simulink model "DSOGI"  (R2018b)
settings: Solver=ode45  StartTime=0.0  StopTime=10.0  MaxStep=0.0001  MinStep=0.00001  RelTol=1e-3
libraries: simulink x1, powerlib_meascontrol x1, powerlib x1
settings Model: Creator=lokes  LastModifiedBy=lokes

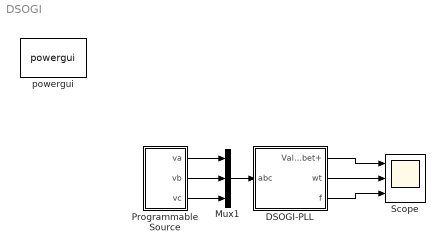
== system DSOGI ==
  DSOGI-PLL : Subsystem
  Mux1 : Mux  Inputs=3
  Programmable Source : Subsystem  mask(DSOGI - PLL){f=50, V=230}
      mask prompts: f "Fundamental grid frequency (f) in Hz"; V "Fundamental grid voltage (V) in RMS volts"
      mask help: Programmable source generates a signal with fundamental and odd harmonic signals upto 13th frequency component.
  Scope : Scope  NumInputPorts=3
  powergui : powerlib/powergui  Priority=1  SimulationMode=Discrete  SampleTime=10e-6  frequency=60  Iterations=50  frequencyindice=60  Pbase=100e6  ErrMax=1e-4  UnitsV=kV  UnitsW=MW  buscounter=0  FunctionMessages=off  echomessages=off  EnableUseOfTLC=off  CurrentSourceSwitches=off  DisableSnubberDevices=off  DisableRonSwitches=off  DisableVfSwitches=off  DisplayEquations=off  SolverType=Tustin/Backward Euler (TBE)  Interpol=off  ExternalGateDelay=off  methode=off  Ts=100  x0status=blocks  SPID=off  SwTol=0  HookPort=off  RestoreLinks=warning  ResistiveCurrentMeasurement=off  Frange=[0:2:500]  Ylog=off  Xlog=on  ShowGrid=off  save=off  variable=ZData  structure=0  ZoomFFT=off  StartTime=0.0  cycles=1  DisplayStyle=1  fundamental=60  FreqAxis=off  MaxFrequency=1000  frequencyindicesteady=1  RmsSteady=1  display=off
  wires:
  Mux1/1 -> DSOGI-PLL/1(abc)
  Programmable Source/1(va) -> Mux1/1
  Programmable Source/2(vb) -> Mux1/2
  Programmable Source/3(vc) -> Mux1/3
  DSOGI-PLL/1(Valp_bet+) -> Scope/1
  DSOGI-PLL/2(wt) -> Scope/2
  DSOGI-PLL/3(f) -> Scope/3

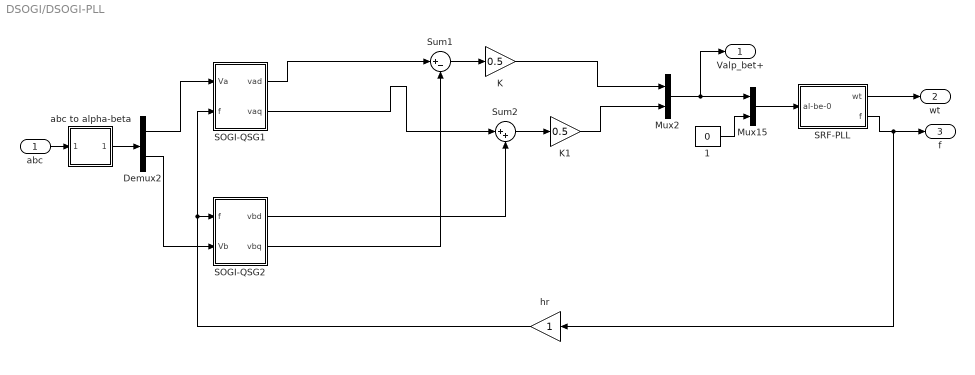
== system DSOGI/DSOGI-PLL ==
  abc : Inport
  1 : Constant  Value=0
  Demux2 : Demux  Outputs=2
  K : Gain  Gain=0.5
  K1 : Gain  Gain=0.5
  Mux15 : Mux  Inputs=2
  Mux2 : Mux  Inputs=2
  SOGI-QSG1 : Subsystem
  SOGI-QSG2 : Subsystem
  SRF-PLL : Subsystem
  Sum1 : Sum  Inputs=|+-
  Sum2 : Sum  Inputs=|++
  abc to alpha-beta : Subsystem
      mask Display:
      | plot([0 1], [0,1])
      | text(0.15,0.7,'abc')
      | text(0.55, 0.3,'\alpha\beta','texmode','on')
  hr : Gain
  Valp_bet+ : Outport
  wt : Outport  Port=2
  f : Outport  Port=3
  wires:
  abc/1 -> abc to alpha-beta/1(abc)
  SOGI-QSG1/1(vad) -> Sum1/1
  Demux2/1 -> SOGI-QSG1/1(Va)
  abc to alpha-beta/1(al_be) -> Demux2/1
  Demux2/2 -> SOGI-QSG2/2(Vb)
  SOGI-QSG2/1(vbd) -> Sum2/2
  SOGI-QSG2/2(vbq) -> Sum1/2
  Sum1/1 -> K/1
  K/1 -> Mux2/1
  SOGI-QSG1/2(vaq) -> Sum2/1
  Sum2/1 -> K1/1
  K1/1 -> Mux2/2
  SRF-PLL/1(wt) -> wt/1
  SRF-PLL/2(f) -> hr/1, f/1
  Mux15/1 -> SRF-PLL/1(al-be-0)
  1/1 -> Mux15/2
  Mux2/1 -> Valp_bet+/1, Mux15/1
  hr/1 -> SOGI-QSG1/2(f), SOGI-QSG2/1(f)

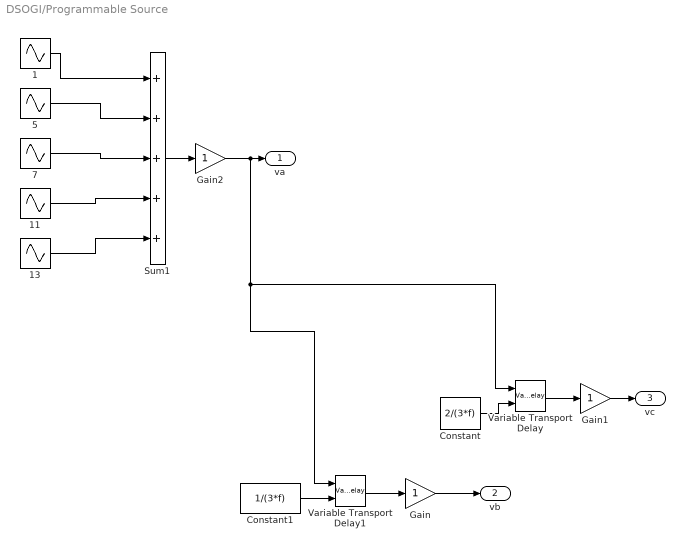
== system DSOGI/Programmable Source ==
  1 : Sin  Amplitude=V*sqrt(2)  Frequency=2*pi*f  Phase=0*pi/2  SampleTime=0
  11 : Sin  Amplitude=V*sqrt(2)/11  Frequency=2*pi*11*f  Phase=0*pi/2  SampleTime=0
  13 : Sin  Amplitude=V*sqrt(2)/13  Frequency=2*pi*13*f  Phase=0*pi/2  SampleTime=0
  5 : Sin  Amplitude=V*sqrt(2)/5  Frequency=2*pi*5*f  Phase=0*pi/2  SampleTime=0
  7 : Sin  Amplitude=V*sqrt(2)/7  Frequency=2*pi*7*f  Phase=0*pi/2  SampleTime=0
  Constant : Constant  Value=2/(3*f)
  Constant1 : Constant  Value=1/(3*f)
  Gain : Gain
  Gain1 : Gain
  Gain2 : Gain
  Sum1 : Sum  Inputs=+++++
  Variable Transport Delay : VariableTransportDelay  VariableDelayType=Variable transport delay  MaximumDelay=10
  Variable Transport Delay1 : VariableTransportDelay  VariableDelayType=Variable transport delay  MaximumDelay=10
  va : Outport
  vb : Outport  Port=2
  vc : Outport  Port=3
  wires:
  Constant1/1 -> Variable Transport Delay1/2
  Constant/1 -> Variable Transport Delay/2
  Variable Transport Delay1/1 -> Gain/1
  Variable Transport Delay/1 -> Gain1/1
  Gain/1 -> vb/1
  Gain1/1 -> vc/1
  Sum1/1 -> Gain2/1
  Gain2/1 -> Variable Transport Delay1/1, Variable Transport Delay/1, va/1
  1/1 -> Sum1/1
  5/1 -> Sum1/2
  7/1 -> Sum1/3
  11/1 -> Sum1/4
  13/1 -> Sum1/5

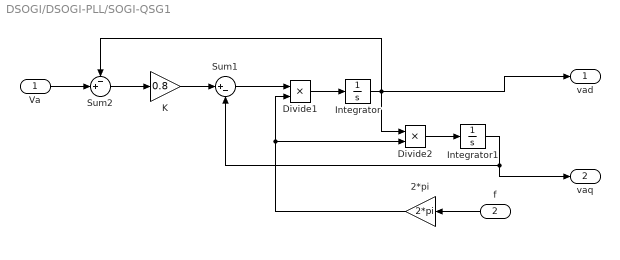
== system DSOGI/DSOGI-PLL/SOGI-QSG1 ==
  Va : Inport
  f : Inport  Port=2
  2*pi : Gain  Gain=2*pi
  Divide1 : Product  Inputs=**
  Divide2 : Product  Inputs=**
  Integrator : Integrator
  Integrator1 : Integrator
  K : Gain  Gain=0.8
  Sum1 : Sum  Inputs=|+-
  Sum2 : Sum  Inputs=-+|
  vad : Outport
  vaq : Outport  Port=2
  wires:
  2*pi/1 -> Divide1/2, Divide2/2
  Va/1 -> Sum2/2
  Integrator1/1 -> vaq/1, Sum1/2
  Divide2/1 -> Integrator1/1
  Integrator/1 -> vad/1, Divide2/1, Sum2/1
  Sum2/1 -> K/1
  K/1 -> Sum1/1
  Sum1/1 -> Divide1/1
  Divide1/1 -> Integrator/1
  f/1 -> 2*pi/1

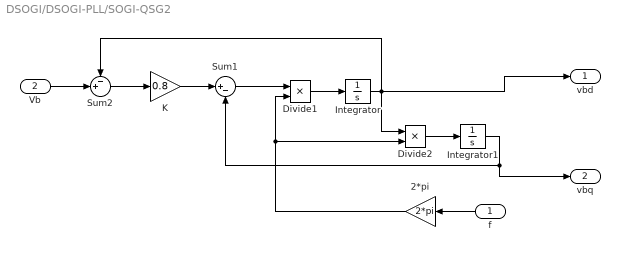
== system DSOGI/DSOGI-PLL/SOGI-QSG2 ==
  f : Inport
  Vb : Inport  Port=2
  2*pi : Gain  Gain=2*pi
  Divide1 : Product  Inputs=**
  Divide2 : Product  Inputs=**
  Integrator : Integrator
  Integrator1 : Integrator
  K : Gain  Gain=0.8
  Sum1 : Sum  Inputs=|+-
  Sum2 : Sum  Inputs=-+|
  vbd : Outport
  vbq : Outport  Port=2
  wires:
  Divide1/1 -> Integrator/1
  Sum1/1 -> Divide1/1
  K/1 -> Sum1/1
  Sum2/1 -> K/1
  Integrator/1 -> Sum2/1, Divide2/1, vbd/1
  Divide2/1 -> Integrator1/1
  Integrator1/1 -> Sum1/2, vbq/1
  Vb/1 -> Sum2/2
  2*pi/1 -> Divide2/2, Divide1/2
  f/1 -> 2*pi/1

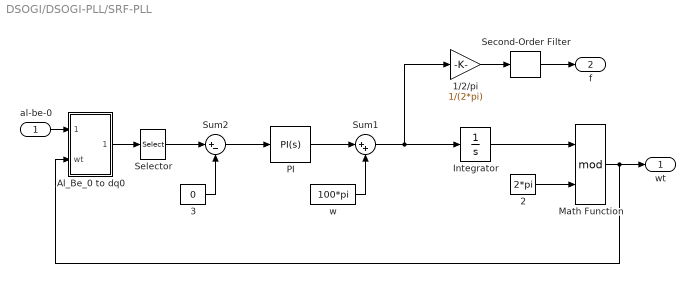
== system DSOGI/DSOGI-PLL/SRF-PLL ==
  al-be-0 : Inport
  1/2/pi : Gain  Gain=1/(2*pi)
  2 : Constant  Value=2*pi
  3 : Constant  Value=0
  Al_Be_0 to dq0 : Subsystem
      mask Display:
      | plot([0 1], [0,1])
      | port_label('input', 1, '\alpha\beta0','texmode','on')
      | port_label('input', 2, 'wt')
      | port_label('output', 1, 'dq0')
  Integrator : Integrator
  Math Function : Math  Operator=mod  SaturateOnIntegerOverflow=on
  "PI " : simulink/Continuous/PID Controller  Controller=PI  Form=Parallel  TimeDomain=Continuous-time  SampleTime=100e-6  IntegratorMethod=Forward Euler  FilterMethod=Forward Euler  ControllerParametersSource=internal  P=10  I=30  D=0  UseFilter=on  N=100  TunerSelectOption=Transfer Function Based (PID Tuner App)  InitialConditionSource=internal  InitialConditionForIntegrator=0  InitialConditionForFilter=0  DifferentiatorICPrevScaledInput=0  ExternalReset=none  TrackingMode=off  Kt=1  LimitOutput=off  UpperSaturationLimit=inf  LowerSaturationLimit=-inf  LinearizeAsGain=on  AntiWindupMode=none  Kb=1  POutMin=[]  POutMax=[]  IOutMin=[]  IOutMax=[]  DOutMin=[]  DOutMax=[]  NOutMin=[]  NOutMax=[]  SumOutMin=[]  SumOutMax=[]  SaturationOutMin=[]  SaturationOutMax=[]  PParamMin=[]  PParamMax=[]  IParamMin=[]  IParamMax=[]  DParamMin=[]  DParamMax=[]  NParamMin=[]  NParamMax=[]  KbParamMin=[]  KbParamMax=[]  KtParamMin=[]  KtParamMax=[]  KbOutMin=[]  KbOutMax=[]  KtOutMin=[]  KtOutMax=[]  IntegratorOutMin=[]  IntegratorOutMax=[]  FilterOutMin=[]  FilterOutMax=[]  SumI1OutMin=[]  SumI1OutMax=[]  SumI2OutMin=[]  SumI2OutMax=[]  SumI3OutMin=[]  SumI3OutMax=[]  SumI4OutMin=[]  SumI4OutMax=[]  SumDOutMin=[]  SumDOutMax=[]  DifferentiatorOutMin=[]  DifferentiatorOutMax=[]  FilterDiffOutCoefMin=[]  FilterDiffOutCoefMax=[]  ReciprocalOutMin=[]  ReciprocalOutMax=[]  SumDenOutMin=[]  SumDenOutMax=[]  SumNumOutMin=[]  SumNumOutMax=[]  DivideOutMin=[]  DivideOutMax=[]  IntegratorContinuousStateAttributes=''  IntegratorStateMustResolveToSignalObject=off  IntegratorRTWStateStorageClass=Auto  FilterContinuousStateAttributes=''  FilterStateMustResolveToSignalObject=off  FilterRTWStateStorageClass=Auto  ParallelPVariant=InternalParameters  IdealPVariant=Disabled  IVariant=InternalParameters  DVariant=Disabled  IntegratorVariant=Continuous  SatVariant=Disabled  AWVariant=Passthrough  PCopyVariant=Disabled  TRVariant=Disabled  FdbkBlocksVariant=Forward  IdealPFdbkVariant=Disabled  SatFdbkVariant=Disabled  DerivativeFilterVariant=Disabled  NVariant=Disabled  NCopyVariant=Disabled_SignalSpec  FilterICVariant=Disabled  IntegratorICVariant=InternalICs  ExternalResetVariant=Disabled  TRSumVariant=Passthrough  SumFdbkVariant=Disabled  SumVariant=Sum_PI
  Second-Order Filter : powerlib_meascontrol/Filters/Second-Order Filter  FilterType=Lowpass  Fo=5  Zeta=0.707  Ts=0  Initialize=off  Vac_Init="[0,  0,  50]"  Vdc_Init=0  PlotResponse=off  FreqRange=[0, 500, 1]
      settings: SourceProductName=Simscape Power Systems  SourceProductBaseCode=PS
  Selector : Selector  InputPortWidth=3  IndexOptions=Index vector (dialog)  Indices=1  OutputSizes=1
  Sum1 : Sum  Inputs=|++
  Sum2 : Sum  Inputs=|+-
  w : Constant  Value=100*pi
  wt : Outport
  f : Outport  Port=2
  wires:
  1/2/pi/1 -> Second-Order Filter/1
  Math Function/1 -> Al_Be_0 to dq0/2(wt), wt/1
  Integrator/1 -> Math Function/1
  2/1 -> Math Function/2
  Sum1/1 -> Integrator/1, 1/2/pi/1
  w/1 -> Sum1/2
  "PI "/1 -> Sum1/1
  Sum2/1 -> "PI "/1
  al-be-0/1 -> Al_Be_0 to dq0/1(Al_Be_0)
  3/1 -> Sum2/2
  Al_Be_0 to dq0/1(dq0) -> Selector/1
  Selector/1 -> Sum2/1
  Second-Order Filter/1 -> f/1

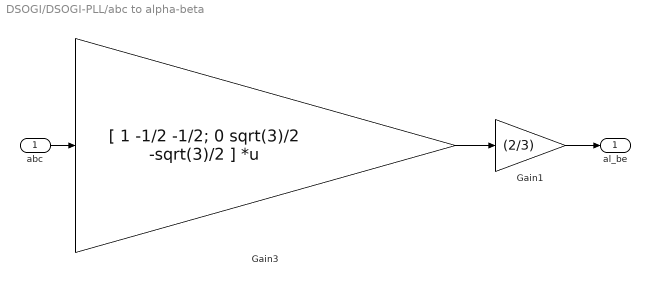
== system DSOGI/DSOGI-PLL/abc to alpha-beta ==
  abc : Inport
  Gain1 : Gain  Gain=(2/3)  SaturateOnIntegerOverflow=on  OutDataTypeStr=Inherit: Same as input  ParamDataTypeStr=Inherit: Same as input
  Gain3 : Gain  Gain="[ 1   -1/2   -1/2; 0   sqrt(3)/2   -sqrt(3)/2 ]"  Multiplication=Matrix(K*u) (u vector)  SaturateOnIntegerOverflow=on  OutDataTypeStr=Inherit: Same as input  ParamDataTypeStr=Inherit: Same as input
  al_be : Outport
  wires:
  abc/1 -> Gain3/1
  Gain1/1 -> al_be/1
  Gain3/1 -> Gain1/1

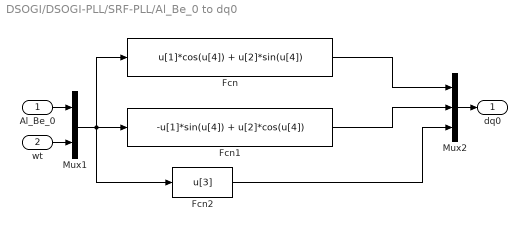
== system DSOGI/DSOGI-PLL/SRF-PLL/Al_Be_0 to dq0 ==
  Al_Be_0 : Inport
  wt : Inport  Port=2
  Fcn : Fcn  Expr=u[1]*cos(u[4]) + u[2]*sin(u[4])
  Fcn1 : Fcn  Expr=-u[1]*sin(u[4]) + u[2]*cos(u[4])
  Fcn2 : Fcn  Expr=u[3]
  Mux1 : Mux  Inputs=[3 1]
  Mux2 : Mux  Inputs=3
  dq0 : Outport
  wires:
  Mux1/1 -> Fcn/1, Fcn2/1, Fcn1/1
  Fcn1/1 -> Mux2/2
  wt/1 -> Mux1/2
  Mux2/1 -> dq0/1
  Al_Be_0/1 -> Mux1/1
  Fcn2/1 -> Mux2/3
  Fcn/1 -> Mux2/1
